simulink model "BattEncThrustRPM"  (R2015b)
settings: Solver=ode4  StartTime=0.0  StopTime=inf  FixedStep=0.05  RelTol=1e-3
values from neighbouring files (symbols this model uses):
  pinvTr = pinv(Tr)    [run_MIP_LQR.m]    (also in run_PendAndHeadingLQR.m; run_Saucer_LQG.m)
libraries: robotlib x13, realtime_pacer_lib x1
settings Model: Creator=saucer  LastModifiedBy=saucer

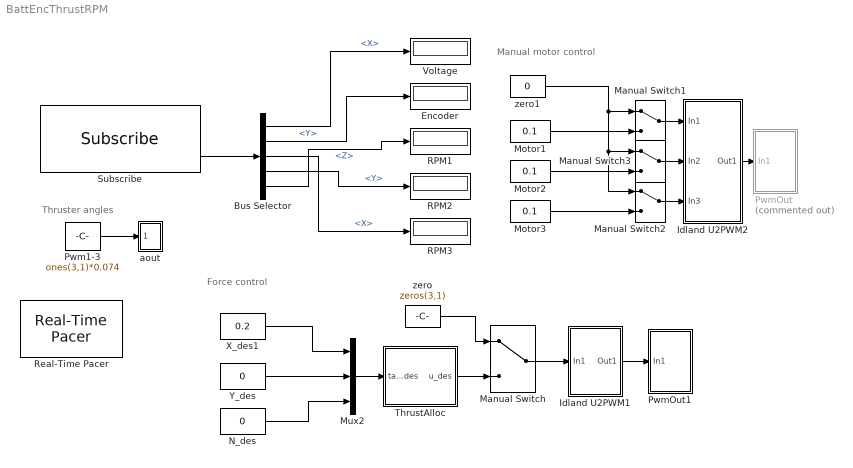
== system BattEncThrustRPM ==
  note: Force control
  note: Manual motor control
  note: Thruster angles
  Bus Selector : BusSelector  OutputSignals=Linear.X,Linear.Y,Angular.X,Angular.Y,Angular.Z
  Encoder : Display
  Idland U2PWM1 : Subsystem
  Idland U2PWM2 : Subsystem
  Manual Switch{,1..3} (4 alike) : ManualSwitch
  Motor1 : Constant  Value=0.1
  Motor2 : Constant  Value=0.1
  Motor3 : Constant  Value=0.1
  Mux2 : Mux  Inputs=3
  N_des : Constant  Value=0
  Pwm1-3 : Constant  Value=ones(3,1)*0.074
  PwmOut : Subsystem  Commented=on
  PwmOut1 : Subsystem
  RPM1 : Display
  RPM2 : Display
  RPM3 : Display
  Real-Time Pacer : realtime_pacer_lib/Real-Time Pacer  simTimePerRealTime=1
  Subscribe : robotlib/Subscribe  SourceLibraryInfo=This block requires Robotics System Toolbox  topicSource=Select from ROS network  topic=/BatterEncoderThrustRPM  messageType=geometry_msgs/Twist  sampleTime=-1  messageQueueLength=1
  ThrustAlloc : Subsystem
  Voltage : Display
  X_des1 : Constant  Value=0.2
  Y_des : Constant  Value=0
  aout : Subsystem
  zero : Constant  Value=zeros(3,1)
  zero1 : Constant  Value=0
  wires:
  Pwm1-3/1 -> aout/1(In1)
  X_des1/1 -> Mux2/1
  Y_des/1 -> Mux2/2
  N_des/1 -> Mux2/3
  Mux2/1 -> ThrustAlloc/1(tau_des)
  zero/1 -> Manual Switch/1
  ThrustAlloc/1(u_des) -> Manual Switch/2
  Idland U2PWM2/1(Out1) -> PwmOut/1(In1)
  Subscribe/2 -> Bus Selector/1
  Bus Selector/1 -> Voltage/1  "<X>"
  Bus Selector/2 -> Encoder/1  "<Y>"
  Bus Selector/4 -> RPM2/1  "<Y>"
  Manual Switch1/1 -> Idland U2PWM2/1(In1)
  Manual Switch2/1 -> Idland U2PWM2/3(In3)
  Manual Switch3/1 -> Idland U2PWM2/2(In2)
  Motor1/1 -> Manual Switch1/2
  Motor2/1 -> Manual Switch3/2
  Motor3/1 -> Manual Switch2/2
  zero1/1 -> Manual Switch1/1, Manual Switch3/1, Manual Switch2/1
  Manual Switch/1 -> Idland U2PWM1/1(In1)
  Idland U2PWM1/1(Out1) -> PwmOut1/1(In1)
  Bus Selector/3 -> RPM3/1  "<X>"
  Bus Selector/5 -> RPM1/1  "<Z>"

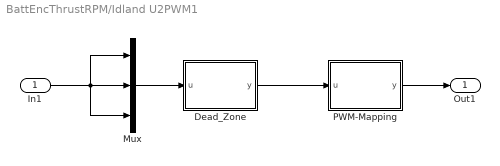
== system BattEncThrustRPM/Idland U2PWM1 ==
  In1 : Inport
  Dead_Zone : MATLAB Function  TreatAsAtomicUnit=on
  Mux : Mux  Inputs=3
  PWM-Mapping : MATLAB Function  TreatAsAtomicUnit=on
  Out1 : Outport
  wires:
  Dead_Zone/1(y) -> PWM-Mapping/1(u)
  In1/1 -> Mux/3, Mux/2, Mux/1
  Mux/1 -> Dead_Zone/1(u)
  PWM-Mapping/1(y) -> Out1/1

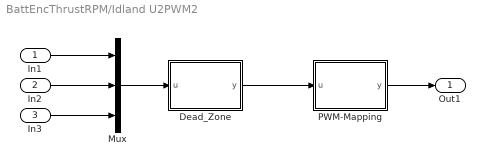
== system BattEncThrustRPM/Idland U2PWM2 ==
  In1 : Inport
  In2 : Inport  Port=2
  In3 : Inport  Port=3
  Dead_Zone : MATLAB Function  TreatAsAtomicUnit=on
  Mux : Mux  Inputs=3
  PWM-Mapping : MATLAB Function  TreatAsAtomicUnit=on
  Out1 : Outport
  wires:
  Dead_Zone/1(y) -> PWM-Mapping/1(u)
  In1/1 -> Mux/1
  Mux/1 -> Dead_Zone/1(u)
  PWM-Mapping/1(y) -> Out1/1
  In2/1 -> Mux/2
  In3/1 -> Mux/3

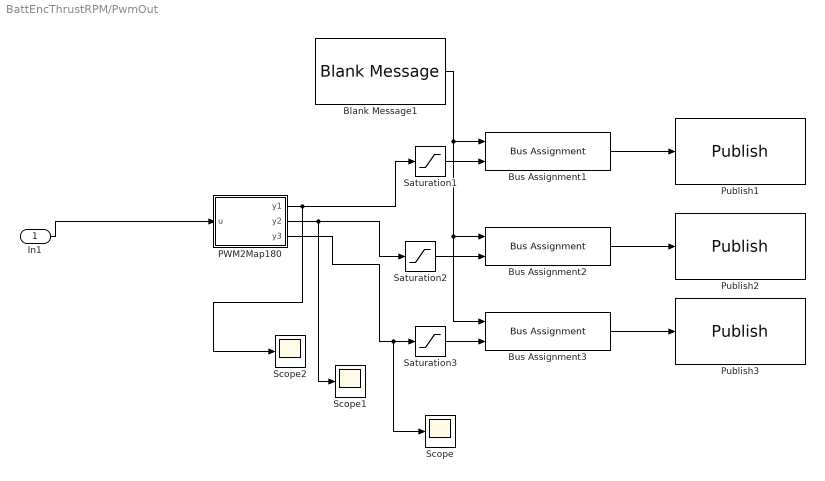
== system BattEncThrustRPM/PwmOut ==
  In1 : Inport
  Blank Message1 : robotlib/Blank Message  SourceLibraryInfo=This block requires Robotics System Toolbox  messageType=std_msgs/UInt16  SampleTime=inf
  Bus Assignment1 : BusAssignment  AssignedSignals=Data
  Bus Assignment2 : BusAssignment  AssignedSignals=Data
  Bus Assignment3 : BusAssignment  AssignedSignals=Data
  "PWM2Map180 " : MATLAB Function  TreatAsAtomicUnit=on
  Publish1 : robotlib/Publish  SourceLibraryInfo=This block requires Robotics System Toolbox  topicSource=Specify your own  topic=/Thrust1  messageType=std_msgs/UInt16  messageQueueLength=1
  Publish2 : robotlib/Publish  SourceLibraryInfo=This block requires Robotics System Toolbox  topicSource=Specify your own  topic=/Thrust2  messageType=std_msgs/UInt16  messageQueueLength=1
  Publish3 : robotlib/Publish  SourceLibraryInfo=This block requires Robotics System Toolbox  topicSource=Specify your own  topic=/Thrust3  messageType=std_msgs/UInt16  messageQueueLength=1
  Saturation1 : Saturate  UpperLimit=170  LowerLimit=10
  Saturation2 : Saturate  UpperLimit=170  LowerLimit=10
  Saturation3 : Saturate  UpperLimit=170  LowerLimit=10
  Scope : Scope
  Scope1 : Scope
  Scope2 : Scope
  wires:
  Bus Assignment3/1 -> Publish3/1
  "PWM2Map180 "/2(y2) -> Saturation2/1, Scope1/1
  Bus Assignment1/1 -> Publish1/1
  Blank Message1/1 -> Bus Assignment3/1, Bus Assignment2/1, Bus Assignment1/1
  In1/1 -> "PWM2Map180 "/1(u)
  "PWM2Map180 "/3(y3) -> Saturation3/1, Scope/1
  "PWM2Map180 "/1(y1) -> Scope2/1, Saturation1/1
  Bus Assignment2/1 -> Publish2/1
  Saturation1/1 -> Bus Assignment1/2
  Saturation2/1 -> Bus Assignment2/2
  Saturation3/1 -> Bus Assignment3/2

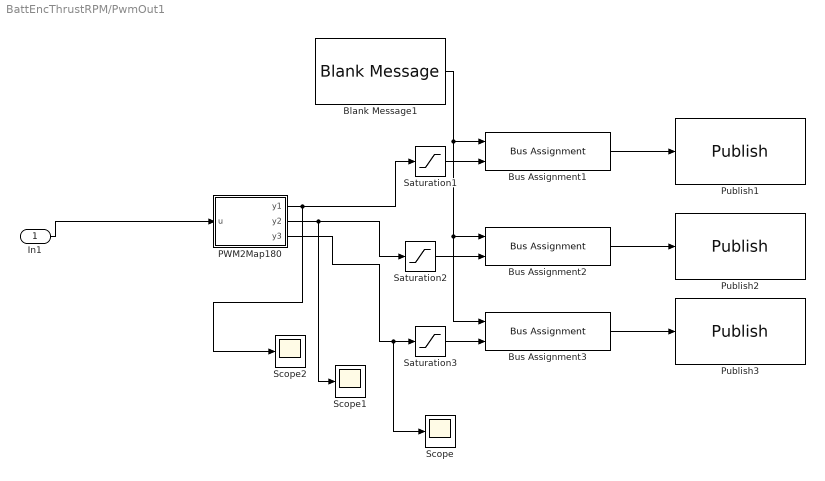
== system BattEncThrustRPM/PwmOut1 ==
  In1 : Inport
  Blank Message1 : robotlib/Blank Message  SourceLibraryInfo=This block requires Robotics System Toolbox  messageType=std_msgs/UInt16  SampleTime=inf
  Bus Assignment1 : BusAssignment  AssignedSignals=Data
  Bus Assignment2 : BusAssignment  AssignedSignals=Data
  Bus Assignment3 : BusAssignment  AssignedSignals=Data
  "PWM2Map180 " : MATLAB Function  TreatAsAtomicUnit=on
  Publish1 : robotlib/Publish  SourceLibraryInfo=This block requires Robotics System Toolbox  topicSource=Specify your own  topic=/Thrust1  messageType=std_msgs/UInt16  messageQueueLength=1
  Publish2 : robotlib/Publish  SourceLibraryInfo=This block requires Robotics System Toolbox  topicSource=Specify your own  topic=/Thrust2  messageType=std_msgs/UInt16  messageQueueLength=1
  Publish3 : robotlib/Publish  SourceLibraryInfo=This block requires Robotics System Toolbox  topicSource=Specify your own  topic=/Thrust3  messageType=std_msgs/UInt16  messageQueueLength=1
  Saturation1 : Saturate  UpperLimit=170  LowerLimit=10
  Saturation2 : Saturate  UpperLimit=170  LowerLimit=10
  Saturation3 : Saturate  UpperLimit=170  LowerLimit=10
  Scope : Scope
  Scope1 : Scope
  Scope2 : Scope
  wires:
  Bus Assignment3/1 -> Publish3/1
  "PWM2Map180 "/2(y2) -> Saturation2/1, Scope1/1
  Bus Assignment1/1 -> Publish1/1
  Blank Message1/1 -> Bus Assignment3/1, Bus Assignment2/1, Bus Assignment1/1
  In1/1 -> "PWM2Map180 "/1(u)
  "PWM2Map180 "/3(y3) -> Saturation3/1, Scope/1
  "PWM2Map180 "/1(y1) -> Scope2/1, Saturation1/1
  Bus Assignment2/1 -> Publish2/1
  Saturation1/1 -> Bus Assignment1/2
  Saturation2/1 -> Bus Assignment2/2
  Saturation3/1 -> Bus Assignment3/2

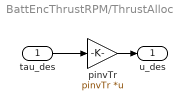
== system BattEncThrustRPM/ThrustAlloc ==
  tau_des : Inport
  pinvTr : Gain  Gain=pinvTr  Multiplication=Matrix(K*u)
  u_des : Outport
  wires:
  pinvTr/1 -> u_des/1
  tau_des/1 -> pinvTr/1

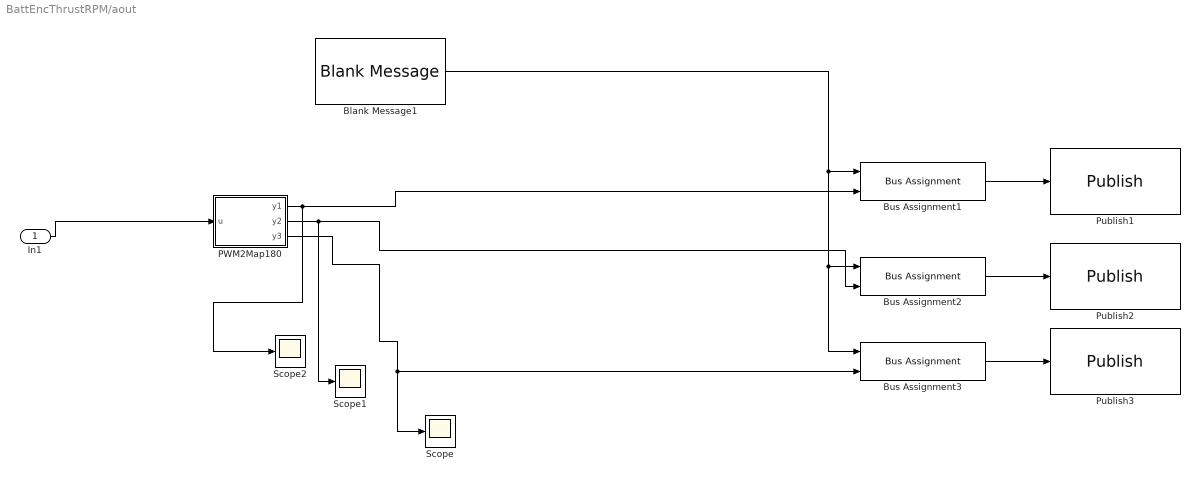
== system BattEncThrustRPM/aout ==
  In1 : Inport
  Blank Message1 : robotlib/Blank Message  SourceLibraryInfo=This block requires Robotics System Toolbox  messageType=std_msgs/UInt16  SampleTime=inf
  Bus Assignment1 : BusAssignment  AssignedSignals=Data
  Bus Assignment2 : BusAssignment  AssignedSignals=Data
  Bus Assignment3 : BusAssignment  AssignedSignals=Data
  "PWM2Map180 " : MATLAB Function  TreatAsAtomicUnit=on
  Publish1 : robotlib/Publish  SourceLibraryInfo=This block requires Robotics System Toolbox  topicSource=Specify your own  topic=/a1  messageType=std_msgs/UInt16  messageQueueLength=1
  Publish2 : robotlib/Publish  SourceLibraryInfo=This block requires Robotics System Toolbox  topicSource=Specify your own  topic=/a2  messageType=std_msgs/UInt16  messageQueueLength=1
  Publish3 : robotlib/Publish  SourceLibraryInfo=This block requires Robotics System Toolbox  topicSource=Specify your own  topic=/a3  messageType=std_msgs/UInt16  messageQueueLength=1
  Scope : Scope
  Scope1 : Scope
  Scope2 : Scope
  wires:
  Bus Assignment2/1 -> Publish2/1
  "PWM2Map180 "/1(y1) -> Bus Assignment1/2, Scope2/1
  "PWM2Map180 "/3(y3) -> Bus Assignment3/2, Scope/1
  In1/1 -> "PWM2Map180 "/1(u)
  Blank Message1/1 -> Bus Assignment1/1, Bus Assignment2/1, Bus Assignment3/1
  Bus Assignment1/1 -> Publish1/1
  "PWM2Map180 "/2(y2) -> Scope1/1, Bus Assignment2/2
  Bus Assignment3/1 -> Publish3/1

== matlab function BattEncThrustRPM/Idland U2PWM1/Dead_Zone ==
  data: u input; y output
function y = fcn(u)
%#codegen
y=[0 ;0 ;0];
for i=1:3
if (u(i)<-0.02);
    y(i)=u(i)*0.8-0.15;
elseif (u(i)>0.02)
    y(i)=u(i)*0.8+0.15;
end
end

== matlab function BattEncThrustRPM/PwmOut/PWM2Map180  ==
  data: u input; y1 output; y2 output; y3 output
function [y1,y2,y3] = fcn(u)
%#codegen
y1=uint16((u(1)-0.027)*180/0.093);
y2=uint16((u(2)-0.027)*180/0.093);
y3=uint16((u(3)-0.027)*180/0.093);

== matlab function BattEncThrustRPM/Idland U2PWM1/PWM-Mapping ==
  data: u input; y output
function y = fcn(u)
y=(u.*0.0255)+(0.0685);
end

== matlab function BattEncThrustRPM/PwmOut1/PWM2Map180  ==
  data: u input; y1 output; y2 output; y3 output
function [y1,y2,y3] = fcn(u)
%#codegen
y1=uint16((u(1)-0.027)*180/0.093);
y2=uint16((u(2)-0.027)*180/0.093);
y3=uint16((u(3)-0.027)*180/0.093);

== matlab function BattEncThrustRPM/aout/PWM2Map180  ==
  data: u input; y1 output; y2 output; y3 output
function [y1,y2,y3] = fcn(u)
%#codegen
y1=uint16((u(1)-0.027)*180/0.093);
y2=uint16((u(2)-0.027)*180/0.093);
y3=uint16((u(3)-0.027)*180/0.093);

== matlab function BattEncThrustRPM/Idland U2PWM2/Dead_Zone ==
  data: u input; y output
function y = fcn(u)
%#codegen
y=[0 ;0 ;0];
for i=1:3
if (u(i)<-0.02);
    y(i)=u(i)*0.8-0.15;
elseif (u(i)>0.02)
    y(i)=u(i)*0.8+0.15;
end
end

== matlab function BattEncThrustRPM/Idland U2PWM2/PWM-Mapping ==
  data: u input; y output
function y = fcn(u)
y=(u.*0.0255)+(0.0685);
end
